simulink model "simulink_armamenti"  (R2025b)
settings: Solver=VariableStepAuto  StartTime=0.0  StopTime=10  RelTol=1e-3
values from neighbouring files (symbols this model uses):
  a = 5    [es4.m]
  b = 8    [es4.m]
  m = 1    [es4.m]
  n = 3    [es4.m]
  r = 2    [es4.m]
  s = 1    [es4.m]
  x0 = [5 12]    [es4.m]
  xmax = 10    [es4.m]
  ymax = 10    [es4.m]
settings Model: Creator=robert  LastModifiedBy=robert

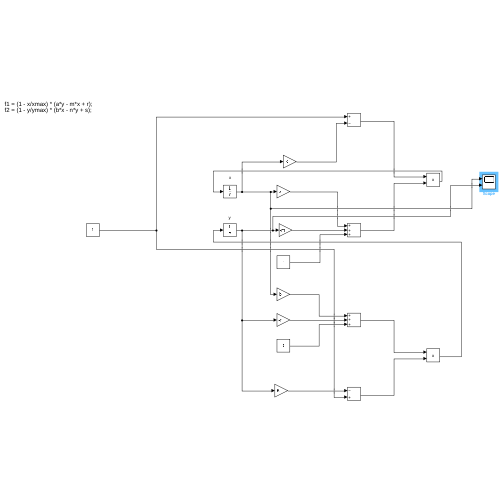
[thumbnail: Simulink's stored preview of the top-level diagram]
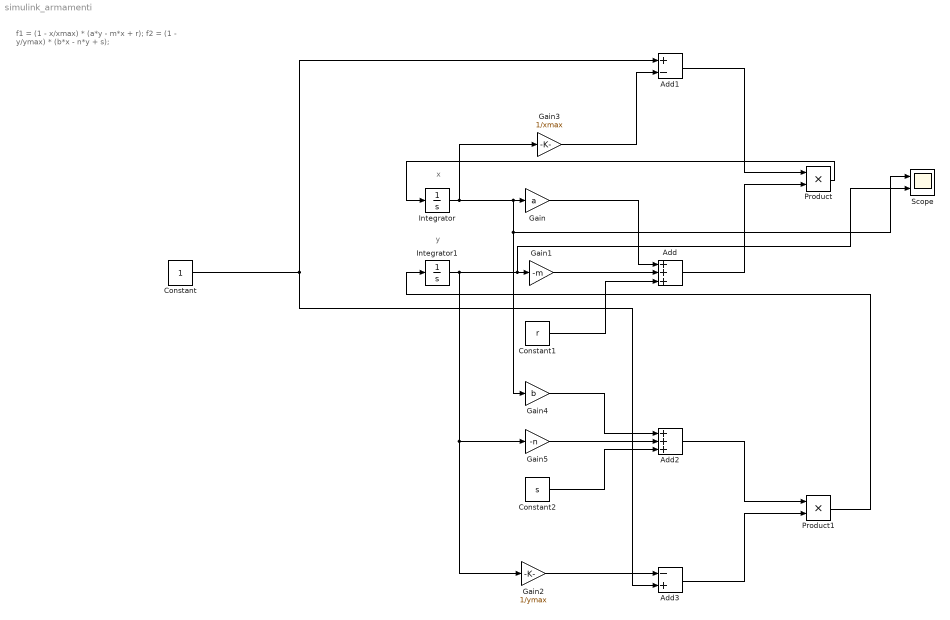
== system simulink_armamenti ==
  note: x
  note: f1 = (1 - x/xmax) * (a*y - m*x + r);
      | f2 = (1 - y/ymax) * (b*x - n*y + s);
  note: y
  Add : Sum  Inputs=+++
  Add1 : Sum  Inputs=+-
  Add2 : Sum  Inputs=+++
  Add3 : Sum  Inputs=-+
  Constant : Constant
  Constant1 : Constant  Value=r
  Constant2 : Constant  Value=s
  Gain : Gain  Gain=a
  Gain1 : Gain  Gain=-m
  Gain2 : Gain  Gain=1/ymax
  Gain3 : Gain  Gain=1/xmax
  Gain4 : Gain  Gain=b
  Gain5 : Gain  Gain=-n
  Integrator : Integrator  InitialCondition=x0(1)
  Integrator1 : Integrator  InitialCondition=x0(2)
  Product : Product
  Product1 : Product
  Scope : Scope  NumInputPorts=2
      settings: ActiveDisplayYMinimum=4.4541337191530692  ActiveDisplayYMaximum=16.922883081317075
  wires:
  Integrator/1 -> Gain3/1, Gain4/1, Scope/1, Gain/1
  Integrator1/1 -> Gain2/1, Gain5/1, Scope/2, Gain1/1
  Gain1/1 -> Add/2
  Gain/1 -> Add/1
  Constant/1 -> Add3/2, Add1/1
  Gain3/1 -> Add1/2
  Add1/1 -> Product/1
  Add/1 -> Product/2
  Product/1 -> Integrator/1
  Constant1/1 -> Add/3
  Gain4/1 -> Add2/1
  Gain5/1 -> Add2/2
  Constant2/1 -> Add2/3
  Add2/1 -> Product1/1
  Add3/1 -> Product1/2
  Product1/1 -> Integrator1/1
  Gain2/1 -> Add3/1
